simulink model "QAM_MatchedFilter"  (R2017b)
settings: Solver=FixedStepDiscrete  StartTime=0.0  StopTime=inf  RelTol=1e-3
libraries: dspmlti4 x2, commrandsrc3 x1, commdigbbndam3 x1, commchan3 x1
settings Model: Creator=rlosada  LastModifiedBy=rlosada
settings SolverCC: AutoInsertRateTranBlk=on
settings DataIOCC: LimitDataPoints=on  SaveOutput=off  SignalLogging=off  SaveTime=off
settings OptimizationCC: LifeSpan=inf  SimCompilerOptimization=on
settings DebuggingCC: AlgebraicLoopMsg=error  SingleTaskRateTransMsg=error  AllowSymbolicDim=off  SFUnexpectedBacktrackingDiag=warning  SFNoUnconditionalDefaultTransitionDiag=warning  SFExecutionAtInitializationDiag=none
settings CodeAppCC: StateflowObjectComments=on
settings GRTTargetCC: TargetLangStandard=C89/C90 (ANSI)  GeneratePreprocessorConditionals=Disable all
settings ConfigComp: CovMetricSettings=dw  CovHtmlReporting=on  CovSaveCumulativeToWorkspaceVar=on  CovSaveSingleToWorkspaceVar=on  CovExternalEMLEnable=off  CovSFcnEnable=off

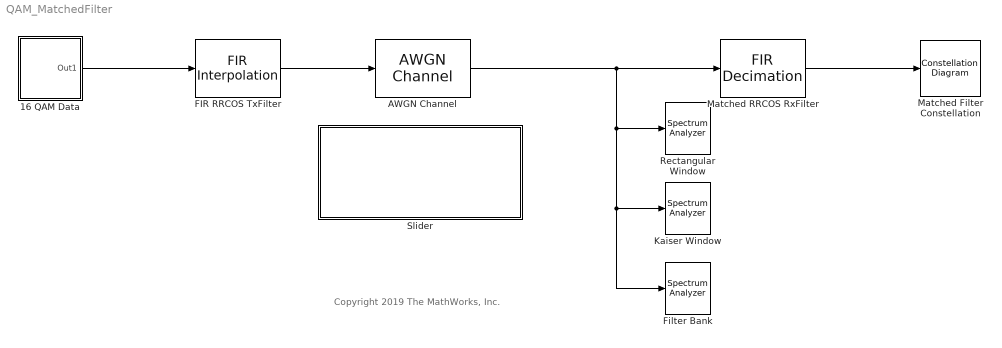
== system QAM_MatchedFilter ==
  note: Copyright 2019 The MathWorks, Inc.
  16 QAM Data : Subsystem
  AWGN Channel : commchan3/AWGN Channel  InputProcessing=Columns as channels (frame based)  seed=67  noiseMode="Signal to noise ratio  (Eb/No)"  EbNodB=84.45467422096317  EsNodB=10  SNRdB=10  bitsPerSym=4  Ps=1  Tsym=16/100e6  variance=1
      settings: SourceProductName=Communications Toolbox
  FIR RRCOS TxFilter : dspmlti4/FIR Interpolation  FilterSource=Dialog parameters  h=rcosdesign(0.45,6, 4,'sqrt')  L=4  FilterObject=FINTERP  InputProcessing=Columns as channels (frame based)  framing=Enforce single-rate processing  outputBufInitCond=0  roundingMode=Floor  overflowMode=off  firstCoeffDataTypeStr=Inherit: Same word length as input  firstCoeffMin=[]  firstCoeffMax=[]  firstCoeffLastDataTypeStr=Inherit: Same word length as input  outputDataTypeStr=Inherit: Same as accumulator  outputMin=[]  outputMax=[]  outputLastDataTypeStr=Inherit: Same as accumulator
      settings: SourceProductName=DSP System Toolbox
  Filter Bank : SpectrumAnalyzer
  Kaiser Window : SpectrumAnalyzer
  Matched RRCOS RxFilter : dspmlti4/FIR Decimation  FilterSource=Dialog parameters  h=rcosdesign(0.45,6, 4,'sqrt')  D=4  filtStruct=Direct form  FilterObject=FDECIM  InputProcessing=Columns as channels (frame based)  framing=Enforce single-rate processing  inputOffset=0  outputBufInitCond=0  roundingMode=Floor  overflowMode=off  firstCoeffDataTypeStr=Inherit: Same word length as input  firstCoeffMin=[]  firstCoeffMax=[]  firstCoeffLastDataTypeStr=Inherit: Same word length as input  outputDataTypeStr=Inherit: Same as accumulator  outputMin=[]  outputMax=[]  outputLastDataTypeStr=Inherit: Same as accumulator
  Matched Filter Constellation : ConstellationDiagram
  Rectangular Window : SpectrumAnalyzer
  Slider : Subsystem  DialogController=hmiCreateDDGDialog  IsWebBlock=on  mask(MWDashboardBlock){webBlockId=a70ff97b-5314-4fe3-ace6-6ab20637aed0, webBlockType=slider, ShowInLibBrowser=on, ShowInitialText=on, HMISrcModelName=QAM_MatchedFilter}
      mask prompts: webBlockId "WebBlock Id"; webBlockType "WebBlock Type"; HMISrcModelName "Source Model"
      mask help: Set value to tune parameters or variables.
      mask Help: helpview([docroot '/mapfiles/simulink.map'], 'hmi_slider')
      mask Display:
      | if strcmp(get_param(bdroot(gcb),'BlockDiagramType'),'library')
      |  image([(matlabroot) '/toolbox/simulink/hmi/icons/Slider.png'])
      | end
  wires:
  16 QAM Data/1(Out1) -> FIR RRCOS TxFilter/1
  FIR RRCOS TxFilter/1 -> AWGN Channel/1
  Matched RRCOS RxFilter/1 -> Matched Filter Constellation/1
  AWGN Channel/1 -> Rectangular Window/1, Kaiser Window/1, Filter Bank/1, Matched RRCOS RxFilter/1

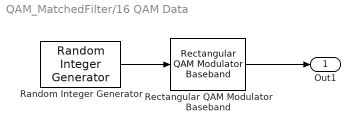
== system QAM_MatchedFilter/16 QAM Data ==
  Random Integer Generator : commrandsrc3/Random Integer Generator  SetSize=16  SeedSource=Auto  Seed=0  SampleTime=1/100e6  SamplesPerFrame=625  OutputDataType=double  SimulateUsing=Code generation
      settings: SourceProductName=Communications Toolbox
  Rectangular QAM Modulator Baseband : commdigbbndam3/Rectangular QAM Modulator Baseband  M=16  InType=Integer  Enc=Gray  Mapping=[0:15]  PowType=Min. distance between symbols  MinDist=2  AvgPow=1  PeakPow=1  Ph=0  outDtype=double  outWordLen=16  outUDDataType=sfix(16)  outFracLenMode=Best precision  outFracLen=15  outDataTypeStr=double  outLastDataTypeStr=double
      settings: SourceProductName=Communications Toolbox
  Out1 : Outport  VectorParamsAs1DForOutWhenUnconnected=on
  wires:
  Random Integer Generator/1 -> Rectangular QAM Modulator Baseband/1
  Rectangular QAM Modulator Baseband/1 -> Out1/1

== system QAM_MatchedFilter/Slider ==
